simulink model "Vent_Drive_Khoo"  (Simulink 7.0)
settings: Solver=ode45  StartTime=0.0  StopTime=10.0  RelTol=1e-3
values from neighbouring files (symbols this model uses):
  DtotalIC = 0.3    [NeuroMuscular_IC.m]    (also in Respiratory_IC.m = 0.32)
  Ic = 45    [Gas_Exchange_IC.m]    (also in Respiratory_IC.m; Vent_Drive_Khoo_IC.m)
  IpCO2 = 38    [Gas_Exchange_IC.m]    (also in Respiratory_IC.m; Vent_Drive_Khoo_IC.m)
  IpO2 = 102.4    [Gas_Exchange_IC.m]    (also in Respiratory_IC.m; Vent_Drive_Khoo_IC.m)
undefined symbols (not defined in the file or in its folder): DAY
libraries: simulink_extras x1
settings Model: Creator=CLM  LastModifiedBy=CLM
settings DebuggingCC: SaveWithParameterizedLinksMsg=none  SignalResolutionControl=TryResolveAllWithWarning  MultiTaskDSMMsg=warning  MultiTaskCondExecSysMsg=none
settings RTWCC: IncludeERTFirstTime=on
settings GRTTargetCC: TargetFcnLib=ansi_tfl_tmw.mat

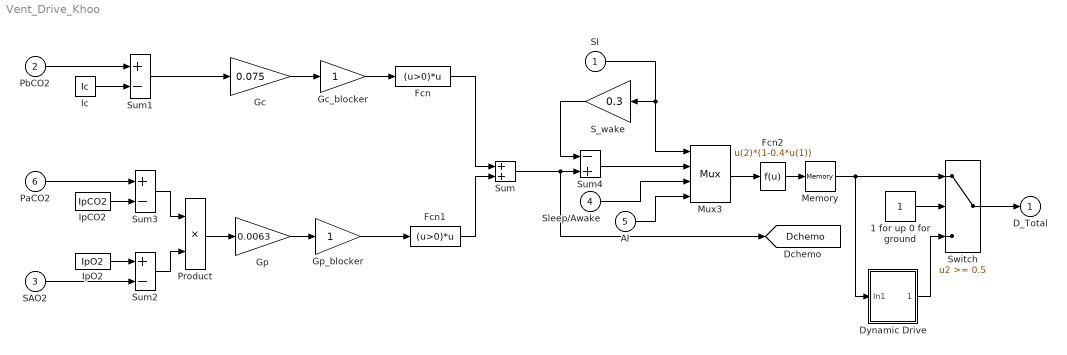
== system Vent_Drive_Khoo ==
  SI : Inport  OutDataType=sfix(16)  OutScaling=2^0
  PbCO2 : Inport  Port=2  OutDataType=sfix(16)  OutScaling=2^0
  SAO2 : Inport  Port=3  OutDataType=sfix(16)  OutScaling=2^0
  Sleep/Awake : Inport  Port=4  OutDataType=sfix(16)  OutScaling=2^0
  AI : Inport  Port=5  OutDataType=sfix(16)  OutScaling=2^0
  PaCO2 : Inport  Port=6  OutDataType=sfix(16)  OutScaling=2^0
  " 1 for up 0 for ground" : Constant  OutDataType=sfix(16)  OutScaling=2^0
  Dynamic Drive : Subsystem
  Fcn : Fcn  Expr=(u>0)*u
  Fcn1 : Fcn  Expr=(u>0)*u
  Fcn2 : Fcn  Expr=u(2)*(1-0.4*u(1))
  Gc : Gain  Gain=0.075  ParameterDataType=sfix(16)  ParameterScaling=2^0  OutDataType=sfix(16)  OutScaling=2^0  SaturateOnIntegerOverflow=on
  Gc_blocker : Gain  ParameterDataType=sfix(16)  ParameterScaling=2^0  OutDataType=sfix(16)  OutScaling=2^0  SaturateOnIntegerOverflow=on
  Gp : Gain  Gain=0.0063  ParameterDataType=sfix(16)  ParameterScaling=2^0  OutDataType=sfix(16)  OutScaling=2^0  SaturateOnIntegerOverflow=on
  Gp_blocker : Gain  ParameterDataType=sfix(16)  ParameterScaling=2^0  OutDataType=sfix(16)  OutScaling=2^0  SaturateOnIntegerOverflow=on
  Ic : Constant  Value=Ic  OutDataType=sfix(16)  OutScaling=2^0
  IpCO2 : Constant  Value=IpCO2  OutDataType=sfix(16)  OutScaling=2^0
  IpO2 : Constant  Value=IpO2  OutDataType=sfix(16)  OutScaling=2^0
  Memory : Memory  X0=DtotalIC
  Mux3 : Mux
  Product : Product  OutDataType=sfix(16)  OutScaling=2^0  SaturateOnIntegerOverflow=on  InputSameDT=on
  S_wake : Gain  Orientation=left  Gain=0.3  ParameterDataType=sfix(16)  ParameterScaling=2^0  OutDataType=sfix(16)  OutScaling=2^0  SaturateOnIntegerOverflow=on
  Sum : Sum  OutDataType=sfix(16)  OutScaling=2^0  SaturateOnIntegerOverflow=on  InputSameDT=on
  Sum1 : Sum  Inputs=+-  OutDataType=sfix(16)  OutScaling=2^0  SaturateOnIntegerOverflow=on  InputSameDT=on
  Sum2 : Sum  Inputs=+-  OutDataType=sfix(16)  OutScaling=2^0  SaturateOnIntegerOverflow=on  InputSameDT=on
  Sum3 : Sum  Inputs=+-  OutDataType=sfix(16)  OutScaling=2^0  SaturateOnIntegerOverflow=on  InputSameDT=on
  Sum4 : Sum  Inputs=-+  OutDataType=sfix(16)  OutScaling=2^0  SaturateOnIntegerOverflow=on  InputSameDT=on
  Switch : Switch  Threshold=0.5  OutDataType=sfix(16)  OutScaling=2^0
  D_Total : Outport  OutDataType=sfix(16)  OutScaling=2^0
  tag scope: Dchemo=global
  wires:
  Gc_blocker/1 -> Fcn/1
  Product/1 -> Gp/1
  Fcn1/1 -> Sum/2
  Fcn/1 -> Sum/1
  SAO2/1 -> Sum2/2
  PaCO2/1 -> Sum3/1
  PbCO2/1 -> Sum1/1
  Ic/1 -> Sum1/2
  IpCO2/1 -> Sum3/2
  IpO2/1 -> Sum2/1
  Gc/1 -> Gc_blocker/1
  Sum1/1 -> Gc/1
  Gp_blocker/1 -> Fcn1/1
  Sum3/1 -> Product/1
  Sum2/1 -> Product/2
  Dynamic Drive/1(Out1) -> Switch/3
  Sum4/1 -> Mux3/2
  Fcn2/1 -> Memory/1
  Mux3/1 -> Fcn2/1
  Sum/1 -> [Dchemo], Sum4/2
  S_wake/1 -> Sum4/1
  Gp/1 -> Gp_blocker/1
  Memory/1 -> Switch/1, Dynamic Drive/1(In1)
  " 1 for up 0 for ground"/1 -> Switch/2
  Switch/1 -> D_Total/1
  Sleep/Awake/1 -> Mux3/3
  AI/1 -> Mux3/4
  SI/1 -> S_wake/1, Mux3/1

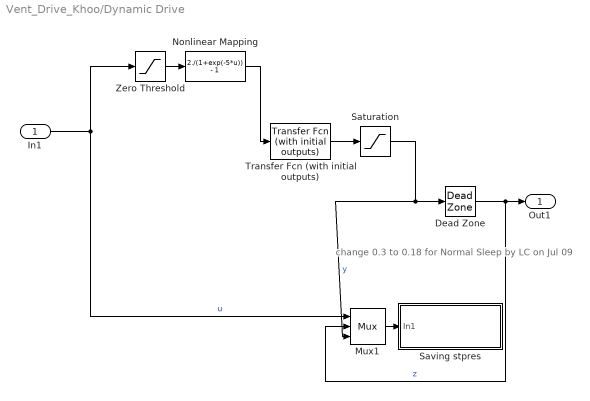
== system Vent_Drive_Khoo/Dynamic Drive ==
  note: change 0.3 to 0.18
      |  for Normal Sleep
      | by LC on Jul 09
  In1 : Inport
  "Dead Zone " : DeadZone  LowerValue=-1000  UpperValue=0.3  SaturateOnIntegerOverflow=on
  Mux1 : Mux  Inputs=3
  Nonlinear Mapping : Fcn  Expr=2./(1+exp(-5*u)) - 1
  Saturation : Saturate  UpperLimit=3  LowerLimit=-1000
  Saving stpres : Subsystem
  Transfer Fcn (with initial outputs) : simulink_extras/Additional Linear/Transfer Fcn (with initial outputs)  SystemSampleTime=-1  N=[20 1]  D=[40 1]  Y0=.35  U0=0.3
  Zero Threshold : Saturate  UpperLimit=1000  LowerLimit=0
  Out1 : Outport
  wires:
  Mux1/1 -> Saving stpres/1(In1)
  "Dead Zone "/1 -> Out1/1, Mux1/2  "z"
  Saturation/1 -> "Dead Zone "/1, Mux1/3  "y"
  Transfer Fcn (with initial outputs)/1 -> Saturation/1
  Zero Threshold/1 -> Nonlinear Mapping/1
  In1/1 -> Zero Threshold/1, Mux1/1  "u"
  Nonlinear Mapping/1 -> Transfer Fcn (with initial outputs)/1

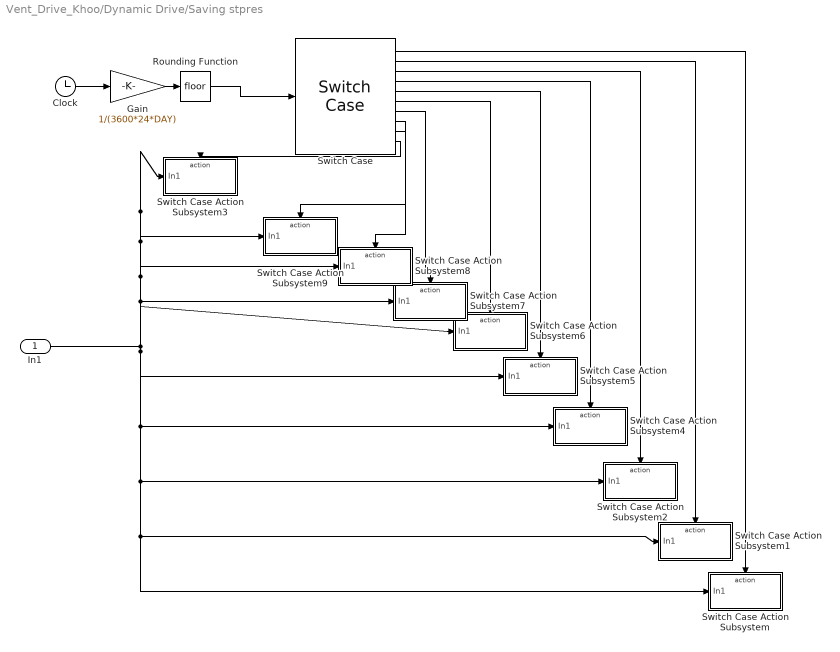
== system Vent_Drive_Khoo/Dynamic Drive/Saving stpres ==
  In1 : Inport  OutDataType=sfix(16)  OutScaling=2^0
  Clock : Clock
      settings: Decimation=10
  Gain : Gain  Gain=1/(3600*24*DAY)  ParameterDataType=sfix(16)  ParameterScaling=2^0  OutDataType=sfix(16)  OutScaling=2^0
  Rounding Function : Rounding
  Switch Case : SwitchCase  CaseConditions={0,1,2,3,4,5,6,7,8}  SampleTime=sampletime
  Switch Case Action Subsystem : Subsystem  TreatAsAtomicUnit=on
  Switch Case Action Subsystem1 : Subsystem  TreatAsAtomicUnit=on
  Switch Case Action Subsystem2 : Subsystem  TreatAsAtomicUnit=on
  Switch Case Action Subsystem3 : Subsystem  TreatAsAtomicUnit=on
  Switch Case Action Subsystem4 : Subsystem  TreatAsAtomicUnit=on
  Switch Case Action Subsystem5 : Subsystem  TreatAsAtomicUnit=on
  Switch Case Action Subsystem6 : Subsystem  TreatAsAtomicUnit=on
  Switch Case Action Subsystem7 : Subsystem  TreatAsAtomicUnit=on
  Switch Case Action Subsystem8 : Subsystem  TreatAsAtomicUnit=on
  Switch Case Action Subsystem9 : Subsystem  TreatAsAtomicUnit=on
  wires:
  Clock/1 -> Gain/1
  Switch Case/1 -> Switch Case Action Subsystem/Action
  Switch Case/2 -> Switch Case Action Subsystem1/Action
  Switch Case/3 -> Switch Case Action Subsystem2/Action
  Switch Case/10 -> Switch Case Action Subsystem3/Action
  Rounding Function/1 -> Switch Case/1
  In1/1 -> Switch Case Action Subsystem/1(In1), Switch Case Action Subsystem1/1(In1), Switch Case Action Subsystem2/1(In1), Switch Case Action Subsystem5/1(In1), Switch Case Action Subsystem3/1(In1), Switch Case Action Subsystem9/1(In1), Switch Case Action Subsystem8/1(In1), Switch Case Action Subsystem7/1(In1), Switch Case Action Subsystem6/1(In1), Switch Case Action Subsystem4/1(In1)
  Gain/1 -> Rounding Function/1
  Switch Case/4 -> Switch Case Action Subsystem4/Action
  Switch Case/5 -> Switch Case Action Subsystem5/Action
  Switch Case/6 -> Switch Case Action Subsystem6/Action
  Switch Case/7 -> Switch Case Action Subsystem7/Action
  Switch Case/8 -> Switch Case Action Subsystem8/Action
  Switch Case/9 -> Switch Case Action Subsystem9/Action

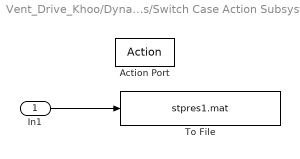
== system Vent_Drive_Khoo/Dynamic Drive/Saving stpres/Switch Case Action Subsystem ==
  In1 : Inport  OutDataType=sfix(16)  OutScaling=2^0
  Action Port : ActionPort
  To File : ToFile  Filename=stpres1.mat  MatrixName=tuzy  SampleTime=sampletime
  wires:
  In1/1 -> To File/1

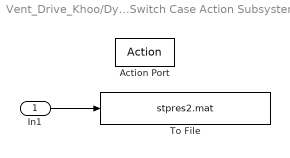
== system Vent_Drive_Khoo/Dynamic Drive/Saving stpres/Switch Case Action Subsystem1 ==
  In1 : Inport  OutDataType=sfix(16)  OutScaling=2^0
  Action Port : ActionPort
  To File : ToFile  Filename=stpres2.mat  MatrixName=tuzy  SampleTime=sampletime
  wires:
  In1/1 -> To File/1

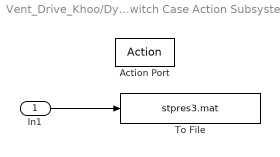
== system Vent_Drive_Khoo/Dynamic Drive/Saving stpres/Switch Case Action Subsystem2 ==
  In1 : Inport  OutDataType=sfix(16)  OutScaling=2^0
  Action Port : ActionPort
  To File : ToFile  Filename=stpres3.mat  MatrixName=tuzy  SampleTime=sampletime
  wires:
  In1/1 -> To File/1

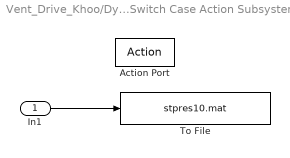
== system Vent_Drive_Khoo/Dynamic Drive/Saving stpres/Switch Case Action Subsystem3 ==
  In1 : Inport  OutDataType=sfix(16)  OutScaling=2^0
  Action Port : ActionPort
  To File : ToFile  Filename=stpres10.mat  MatrixName=tuzy  SampleTime=sampletime
  wires:
  In1/1 -> To File/1

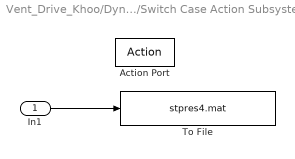
== system Vent_Drive_Khoo/Dynamic Drive/Saving stpres/Switch Case Action Subsystem4 ==
  In1 : Inport  OutDataType=sfix(16)  OutScaling=2^0
  Action Port : ActionPort
  To File : ToFile  Filename=stpres4.mat  MatrixName=tuzy  SampleTime=sampletime
  wires:
  In1/1 -> To File/1

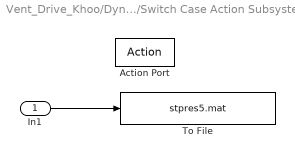
== system Vent_Drive_Khoo/Dynamic Drive/Saving stpres/Switch Case Action Subsystem5 ==
  In1 : Inport  OutDataType=sfix(16)  OutScaling=2^0
  Action Port : ActionPort
  To File : ToFile  Filename=stpres5.mat  MatrixName=tuzy  SampleTime=sampletime
  wires:
  In1/1 -> To File/1

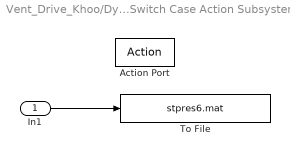
== system Vent_Drive_Khoo/Dynamic Drive/Saving stpres/Switch Case Action Subsystem6 ==
  In1 : Inport  OutDataType=sfix(16)  OutScaling=2^0
  Action Port : ActionPort
  To File : ToFile  Filename=stpres6.mat  MatrixName=tuzy  SampleTime=sampletime
  wires:
  In1/1 -> To File/1

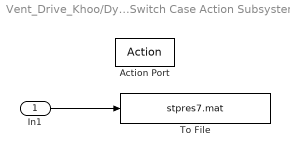
== system Vent_Drive_Khoo/Dynamic Drive/Saving stpres/Switch Case Action Subsystem7 ==
  In1 : Inport  OutDataType=sfix(16)  OutScaling=2^0
  Action Port : ActionPort
  To File : ToFile  Filename=stpres7.mat  MatrixName=tuzy  SampleTime=sampletime
  wires:
  In1/1 -> To File/1

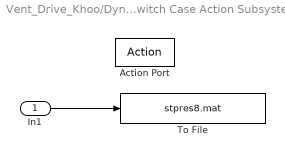
== system Vent_Drive_Khoo/Dynamic Drive/Saving stpres/Switch Case Action Subsystem8 ==
  In1 : Inport  OutDataType=sfix(16)  OutScaling=2^0
  Action Port : ActionPort
  To File : ToFile  Filename=stpres8.mat  MatrixName=tuzy  SampleTime=sampletime
  wires:
  In1/1 -> To File/1

== system Vent_Drive_Khoo/Dynamic Drive/Saving stpres/Switch Case Action Subsystem9 ==
  In1 : Inport  OutDataType=sfix(16)  OutScaling=2^0
  Action Port : ActionPort
  To File : ToFile  Filename=stpres9.mat  MatrixName=tuzy  SampleTime=sampletime
  wires:
  In1/1 -> To File/1
